simulink model "MSE_PLANT"  (R2025b)
settings: Solver=ode4  StartTime=0.0  StopTime=7  FixedStep=T  RelTol=1e-3  EnableMultiTasking=on
values from neighbouring files (symbols this model uses):
  b_sim = 0    [lab_1.m]    (also in lab_3.m)
  k_sim = 0    [lab_1.m]    (also in lab_3.m)
  Kt = Kt*motor_eff    (= 0.028)    [lab_1.m]    (also in lab_3.m)
  r = 0.01    [lab_1.m]    (also in lab_3.m)
  T = 0.001    [lab_1.m]    (also in lab_3.m)
undefined symbols (not defined in the file or in its folder): K_switch, Kd, Ki, Kp, National_Instruments, PCIe
libraries: sldrtlib x5, slpidlib x1
settings Model: ModifiedByFormat=C. Gokcek  SimulationMode=external  ExtModeTrigDuration=50  ExtModeWriteAllDataToWs=on  Creator=fdepi  LastModifiedBy=C. Gokcek
settings SolverCC: AlgebraicLoopSolver=TrustRegion
settings DataIOCC: SaveFormat=Array  SaveOutput=off  SignalLogging=off  DSMLogging=off  SaveTime=off  ReturnWorkspaceOutputs=off
settings OptimizationCC: ReuseModelBlockBuffer=off  ExpressionDepthLimit=2147483647.0  InitFltsAndDblsToZero=on  EfficientMapNaN2IntZero=off  LifeSpan=inf  SimCompilerOptimization=on
settings DebuggingCC: UnderspecifiedInitializationDetection=Classic  MergeDetectMultiDrivingBlocksExec=none  UnconnectedInputMsg=warning  UnconnectedOutputMsg=warning  UnconnectedLineMsg=warning  AllowSymbolicDim=off  StateNameClashWarn=warning  SFUnexpectedBacktrackingDiag=warning  SFNoUnconditionalDefaultTransitionDiag=warning  SFExecutionAtInitializationDiag=none  ArithmeticOperatorsInVariantConditions=warning
settings HardwareCC: ProdBitPerLong=64.0  ProdHWDeviceType=Intel->x86-64 (Linux 64)  TargetBitPerLong=64.0  TargetBitPerPointer=64.0  TargetIntDivRoundTo=Zero  TargetEndianess=LittleEndian  TargetWordSize=64.0  TargetHWDeviceType=Intel->x86-64
settings ModelReferenceCC: EnableRefExpFcnMdlSchedulingChecks=on  PropagateSignalLabelsOutOfModel=off
settings SFSimCC: SimUseLocalCustomCode=off  CustomCodeUndefinedFunction=UseInterfaceOnly
settings RTWCC: SystemTargetFile=sldrt.tlc  TemplateMakefile=sldrt.tmf  RTWVerbose=off  TLCAssert=on  RTWUseLocalCustomCode=off  RTWCompilerOptimization=on  GPUComputeCapability=3.5  DLArmComputeVersion=19.05  Description=Simulink Desktop Real-Time
settings CodeAppCC: GenerateComments=off  MaxIdLength=95.0  SimulinkBlockComments=off
settings SimulinkDesktopRealTimeCC: ExtModeTransport=0.0  ExtModeStaticAllocSize=1000000.0  TargetLibSuffix=_sldrt.a  TargetPreCompLibLocation=C:\Program Files\MATLAB\R2025b\toolbox\sldrt\lib\win64  TargetLangStandard=C89/C90 (ANSI)  MultiwordLength=2048.0  DynamicStringBufferSize=256.0  ParMdlRefBuildCompliant=on  PreserveMATLABNamespacesInGeneratedCode=on  SubcomponentCodeInterfacePackaging=Reusable function  SupportVariableSizeSignals=off
settings ConfigComp: CovMetricSettings=dw  CovSaveCumulativeToWorkspaceVar=on  CovSaveSingleToWorkspaceVar=on  CovExternalEMLEnable=off  CovSFcnEnable=off

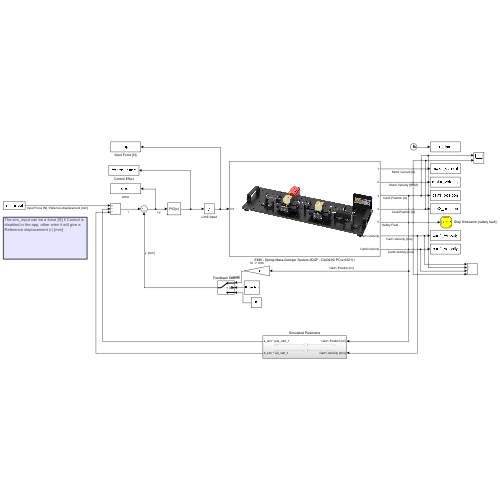
[thumbnail: Simulink's stored preview of the top-level diagram]
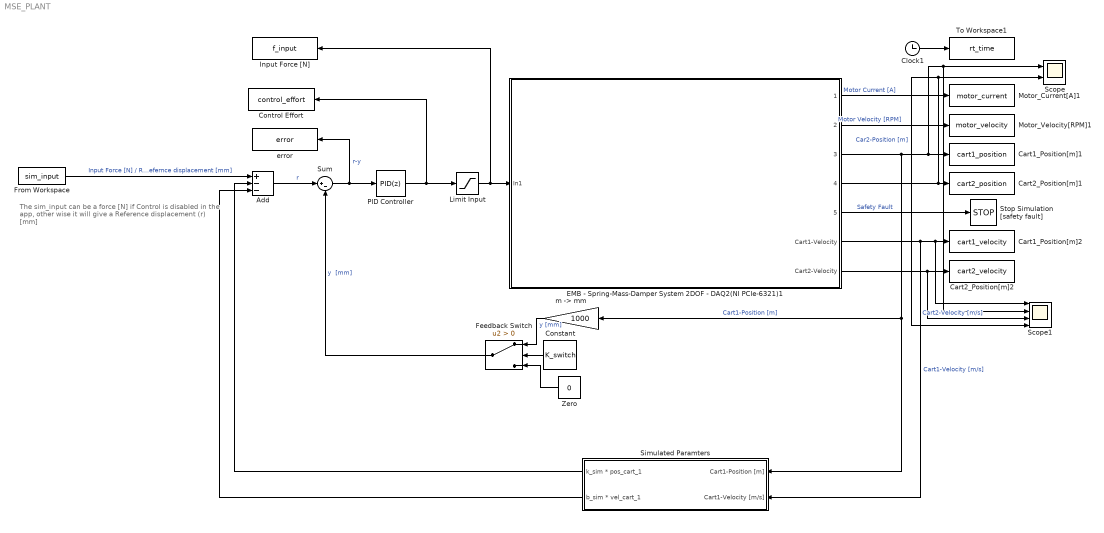
== system MSE_PLANT ==
  note: The sim_input can be a force [N] if Control is
      | disabled in the app, other wise it will give a
      | Reference displacement (r) [mm]
  Add : Sum  Inputs=+--
  Cart1_Position[m]1 : ToWorkspace  VariableName=cart1_position  SampleTime=-1
  Cart1_Position[m]2 : ToWorkspace  VariableName=cart1_velocity  SampleTime=-1
  Cart2_Position[m]1 : ToWorkspace  VariableName=cart2_position  SampleTime=-1
  Cart2_Position[m]2 : ToWorkspace  VariableName=cart2_velocity  SampleTime=-1
  Clock1 : Clock
  Constant : Constant  Value=K_switch
  Control Effort : ToWorkspace  VariableName=control_effort  SampleTime=-1
  EMB - Spring-Mass-Damper System 2DOF - DAQ2(NI PCIe-6321)1 : Subsystem
      mask Display: image('EMB-SMDS-2DOF.png');
  Feedback Switch : Switch  Criteria=u2 > Threshold  SaturateOnIntegerOverflow=off  InputSameDT=off
  From Workspace : FromWorkspace  VariableName=sim_input
  Input Force [N] : ToWorkspace  VariableName=f_input  SampleTime=-1
  Limit Input : Saturate  UpperLimit=10  LowerLimit=-10
  Motor_Current[A]1 : ToWorkspace  VariableName=motor_current  SampleTime=-1
  Motor_Velocity[RPM]1 : ToWorkspace  VariableName=motor_velocity  SampleTime=-1
  PID Controller : slpidlib/PID Controller  Controller=PID  Form=Parallel  TimeDomain=Discrete-time  UseExternalTs=off  SampleTime=T  IntegratorMethod=Forward Euler  FilterMethod=Forward Euler  ControllerParametersSource=internal  P=Kp  I=Ki  UseKiTs=off  D=Kd  UseExternalDerivativeSource=off  N=100  UseFilter=on  TunerSelectOption=Transfer Function Based (PID Tuner App)  InitialConditionSource=internal  InitialConditionForIntegrator=0  InitialConditionForFilter=0  DifferentiatorICPrevScaledInput=0  ExternalReset=none  TrackingMode=off  Kt=1  LimitOutput=off  SatLimitsSource=internal  UpperSaturationLimit=inf  LowerSaturationLimit=-inf  LinearizeAsGain=on  AntiWindupMode=none  Kb=1  LimitIntegrator=off  UpperIntegratorSaturationLimit=inf  LowerIntegratorSaturationLimit=-inf  POutMin=[]  POutMax=[]  IOutMin=[]  IOutMax=[]  DOutMin=[]  DOutMax=[]  NOutMin=[]  NOutMax=[]  SumOutMin=[]  SumOutMax=[]  SaturationOutMin=[]  SaturationOutMax=[]  PParamMin=[]  PParamMax=[]  IParamMin=[]  IParamMax=[]  DParamMin=[]  DParamMax=[]  NParamMin=[]  NParamMax=[]  KbParamMin=[]  KbParamMax=[]  KtParamMin=[]  KtParamMax=[]  KbOutMin=[]  KbOutMax=[]  KtOutMin=[]  KtOutMax=[]  IntegratorOutMin=[]  IntegratorOutMax=[]  FilterOutMin=[]  FilterOutMax=[]  SumI1OutMin=[]  SumI1OutMax=[]  SumI2OutMin=[]  SumI2OutMax=[]  SumI3OutMin=[]  SumI3OutMax=[]  SumI4OutMin=[]  SumI4OutMax=[]  SumDOutMin=[]  SumDOutMax=[]  DifferentiatorOutMin=[]  DifferentiatorOutMax=[]  FilterDiffOutCoefMin=[]  FilterDiffOutCoefMax=[]  ReciprocalOutMin=[]  ReciprocalOutMax=[]  SumDenOutMin=[]  SumDenOutMax=[]  SumNumOutMin=[]  SumNumOutMax=[]  DivideOutMin=[]  DivideOutMax=[]  UdiffTsProdOutMin=[]  UdiffTsProdOutMax=[]  NTsProdOutMin=[]  NTsProdOutMax=[]  UintegralTsProdOutMin=[]  UintegralTsProdOutMax=[]  UngainTsProdOutMin=[]  UngainTsProdOutMax=[]  ClampingZeroOutDataTypeStr=Inherit: Inherit via back propagation  ClampingZeroOutMin=[]  ClampingZeroOutMax=[]  FilterDenConstantOutDataTypeStr=Inherit: Inherit via back propagation  FilterDenConstantOutMin=[]  FilterDenConstantOutMax=[]  PCopyOutDataTypeStr=Inherit: Inherit via back propagation  PCopyOutMin=[]  PCopyOutMax=[]  NCopyOutDataTypeStr=Inherit: Inherit via back propagation  NCopyOutMin=[]  NCopyOutMax=[]  IntegratorContinuousStateAttributes=''  IntegratorStateMustResolveToSignalObject=off  IntegratorRTWStateStorageClass=Auto  FilterContinuousStateAttributes=''  FilterStateMustResolveToSignalObject=off  FilterRTWStateStorageClass=Auto  ParallelPVariant=InternalParameters  IdealPVariant=Disabled  IVariant=InternalParameters  DVariant=InternalParameters  IntegratorVariant=Discrete  SatVariant=Disabled  AWVariant=Passthrough  PCopyVariant=Disabled  TRVariant=Disabled  FdbkBlocksVariant=Forward  IdealPFdbkVariant=Disabled  SatFdbkVariant=Disabled  DerivativeFilterVariant=ForwardEulerFilter  NVariant=InternalParameters  NCopyVariant=Disabled  FilterICVariant=InternalICsFilter  IntegratorICVariant=InternalICs  ExternalResetVariant=Disabled  TRSumVariant=Passthrough  SumFdbkVariant=Disabled  SumVariant=Sum_PID  TsampFilterVariant=InternalTs  TsampNgainVariant=Passthrough  TsampIntegralVariant=Disabled_SignalSpec  ExternalSaturationOutDataTypeStr=Inherit: Same as second input  DerivativeSourceVariant=ErrorSignal  PreIntVariant=InternalPreInt
  Scope : Scope  NumInputPorts=2
      settings: ActiveDisplayYMinimum=-0.026393909411938546  ActiveDisplayYMaximum=0.050293861298803644
  Scope1 : Scope  NumInputPorts=4
      settings: ActiveDisplayYMinimum=-0.025542874999999996  ActiveDisplayYMaximum=0.029194124999999994
  Simulated Paramters : Subsystem
  Stop Simulation [safety fault] : Stop
  Sum : Sum  Inputs=|+-
  To Workspace1 : ToWorkspace  VariableName=rt_time  SampleTime=-1
  Zero : Constant  Value=0  OutDataTypeStr=Inherit: Inherit via back propagation
  error : ToWorkspace  VariableName=error  SampleTime=-1
  "m -> mm" : Gain  Gain=1000
  wires:
  EMB - Spring-Mass-Damper System 2DOF - DAQ2(NI PCIe-6321)1/7(Cart2-Velocity) -> Scope1/3, Cart2_Position[m]2/1  "Cart2-Velocity [m/s]"
  EMB - Spring-Mass-Damper System 2DOF - DAQ2(NI PCIe-6321)1/6(Cart1-Velocity) -> Simulated Paramters/2(Cart1-Velocity [m/s]), Scope1/1, Cart1_Position[m]2/1  "Cart1-Velocity [m/s]"
  EMB - Spring-Mass-Damper System 2DOF - DAQ2(NI PCIe-6321)1/1(1) -> Motor_Current[A]1/1  "Motor Current [A]"
  EMB - Spring-Mass-Damper System 2DOF - DAQ2(NI PCIe-6321)1/3(3) -> Simulated Paramters/1(Cart1-Position [m]), "m -> mm"/1, Scope/1, Scope1/2, Cart1_Position[m]1/1  "Cart1-Position [m]"
  EMB - Spring-Mass-Damper System 2DOF - DAQ2(NI PCIe-6321)1/2(2) -> Motor_Velocity[RPM]1/1  "Motor Velocity [RPM]"
  Limit Input/1 -> Input Force [N]/1, EMB - Spring-Mass-Damper System 2DOF - DAQ2(NI PCIe-6321)1/1(In1)
  EMB - Spring-Mass-Damper System 2DOF - DAQ2(NI PCIe-6321)1/5(5) -> Stop Simulation [safety fault]/1  "Safety Fault"
  EMB - Spring-Mass-Damper System 2DOF - DAQ2(NI PCIe-6321)1/4(4) -> Scope/2, Scope1/4, Cart2_Position[m]1/1  "Car2-Position [m]"
  Clock1/1 -> To Workspace1/1
  From Workspace/1 -> Add/1  "Input Force [N] / Refernce displacement [mm]"
  Simulated Paramters/1(k_sim * pos_cart_1) -> Add/2
  Simulated Paramters/2(b_sim * vel_cart_1) -> Add/3
  Zero/1 -> Feedback Switch/3
  "m -> mm"/1 -> Feedback Switch/1  "y [mm]"
  Add/1 -> Sum/1  "r"
  Sum/1 -> error/1, PID Controller/1  "r-y"
  PID Controller/1 -> Control Effort/1, Limit Input/1
  Feedback Switch/1 -> Sum/2  "y  [mm]"
  Constant/1 -> Feedback Switch/2

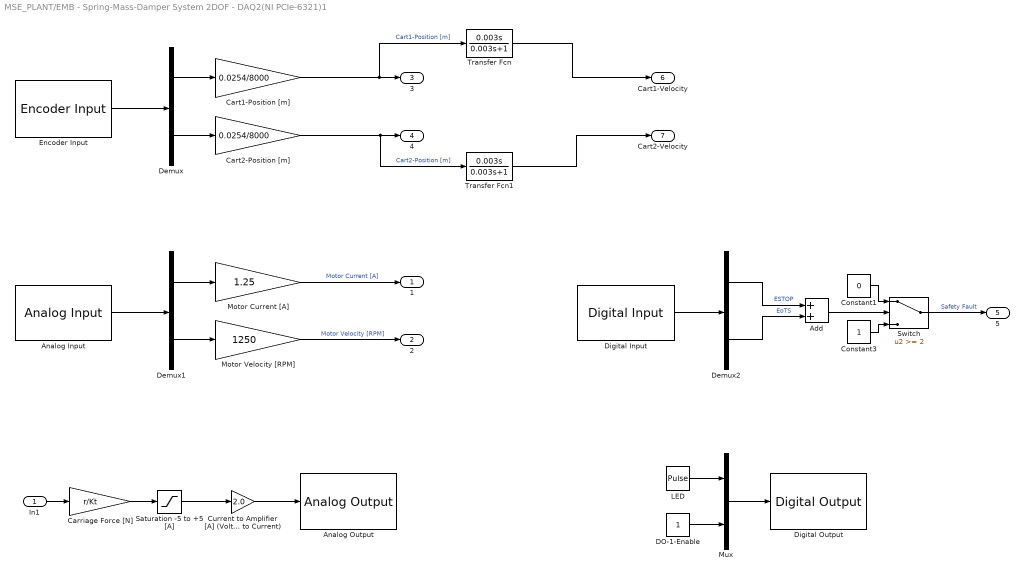
== system MSE_PLANT/EMB - Spring-Mass-Damper System 2DOF - DAQ2(NI PCIe-6321)1 ==
  In1 : Inport
  Add : Sum
  Analog Input : sldrtlib/Analog Input  SampleTime=T  MaxMissedTicks=10  ShowMissedTicks=off  YieldWhenWaiting=off  DrvName=National_Instruments/PCIe-6321  DrvAddress=4294967295  DrvOptions=[0 15 0 2 2 2 2]  Channels=[1,2]  RangeMode=1  VoltRange=2  DataType=1
      settings: AttributesFormatString=National Instruments\nPCIe-6321 [auto]
  Analog Output : sldrtlib/Analog Output  SampleTime=T  MaxMissedTicks=10  ShowMissedTicks=off  YieldWhenWaiting=off  DrvName=National_Instruments/PCIe-6321  DrvAddress=4294967295  DrvOptions=[0 15 0 2 2 2 2]  Channels=[1]  RangeMode=1  VoltRange=1  InitialValue=0  FinalValue=0
      settings: AttributesFormatString=National Instruments\nPCIe-6321 [auto]
  Carriage Force [N] : Gain  Gain=r/Kt
  Cart1-Position [m] : Gain  Gain=0.0254/8000
  Cart2-Position [m] : Gain  Gain=0.0254/8000
  Constant1 : Constant  Value=0
  Constant3 : Constant
  Current to Amplifier [A] (Voltage to Current) : Gain  Gain=2.0
  DO-1-Enable : Constant  OutDataTypeStr=double
  Demux : Demux  Outputs=2
  Demux1 : Demux  Outputs=2
  Demux2 : Demux  Outputs=2
  Digital Input : sldrtlib/Digital Input  SampleTime=T  MaxMissedTicks=10  ShowMissedTicks=off  YieldWhenWaiting=off  DrvName=National_Instruments/PCIe-6321  DrvAddress=4294967295  DrvOptions=[0 15 0 2 2 2 2]  Channels=[5,6]  BitMode=1  DataType=1
      settings: AttributesFormatString=National Instruments\nPCIe-6321 [auto]
  Digital Output : sldrtlib/Digital Output  SampleTime=T  MaxMissedTicks=10  ShowMissedTicks=off  YieldWhenWaiting=off  DrvName=National_Instruments/PCIe-6321  DrvAddress=4294967295  DrvOptions=[0 15 0 2 2 2 2]  Channels=[1,2]  BitMode=1  InitialValue=0  FinalValue=0
      settings: AttributesFormatString=National Instruments\nPCIe-6321 [auto]
  Encoder Input : sldrtlib/Encoder Input  SampleTime=T  MaxMissedTicks=10  ShowMissedTicks=off  YieldWhenWaiting=off  DrvName=National_Instruments/PCIe-6321  DrvAddress=4294967295  DrvOptions=[0 15 0 2 2 2 2]  Channels=[1,2]  QuadMode=3  IndexPulse=1  InputFilter=Inf  DataType=1
      settings: AttributesFormatString=National Instruments\nPCIe-6321 [auto]
  LED : DiscretePulseGenerator  PulseType=Time based  Period=0.5  PulseWidth=50
  Motor Current [A] : Gain  Gain=1.25
  Motor Velocity [RPM] : Gain  Gain=1250
  Mux : Mux  Inputs=2
  Saturation -5 to +5 [A] : Saturate  UpperLimit=5  LowerLimit=-5
  Switch : Switch  Threshold=2  SaturateOnIntegerOverflow=off  InputSameDT=off
  Transfer Fcn : TransferFcn  Numerator=[0.003 0]  Denominator=[0.003 1]
  Transfer Fcn1 : TransferFcn  Numerator=[0.003 0]  Denominator=[0.003 1]
  1 : Outport
  2 : Outport  Port=2
  3 : Outport  Port=3
  4 : Outport  Port=4
  5 : Outport  Port=5
  Cart1-Velocity : Outport  Port=6
  Cart2-Velocity : Outport  Port=7
  wires:
  Current to Amplifier [A] (Voltage to Current)/1 -> Analog Output/1
  Constant1/1 -> Switch/1
  Constant3/1 -> Switch/3
  DO-1-Enable/1 -> Mux/2
  Carriage Force [N]/1 -> Saturation -5 to +5 [A]/1
  Mux/1 -> Digital Output/1
  Motor Current [A]/1 -> 1/1  "Motor Current [A]"
  Cart1-Position [m]/1 -> Transfer Fcn/1, 3/1  "Cart1-Position [m]"
  Encoder Input/1 -> Demux/1
  Switch/1 -> 5/1  "Safety Fault"
  Demux1/2 -> Motor Velocity [RPM]/1
  Demux/2 -> Cart2-Position [m]/1
  Saturation -5 to +5 [A]/1 -> Current to Amplifier [A] (Voltage to Current)/1
  Demux1/1 -> Motor Current [A]/1
  Motor Velocity [RPM]/1 -> 2/1  "Motor Velocity [RPM]"
  Demux2/2 -> Add/2  "EoTS"
  Demux/1 -> Cart1-Position [m]/1
  Digital Input/1 -> Demux2/1
  Demux2/1 -> Add/1  "ESTOP"
  Analog Input/1 -> Demux1/1
  LED/1 -> Mux/1
  Add/1 -> Switch/2
  In1/1 -> Carriage Force [N]/1
  Cart2-Position [m]/1 -> Transfer Fcn1/1, 4/1  "Cart2-Position [m]"
  Transfer Fcn/1 -> Cart1-Velocity/1
  Transfer Fcn1/1 -> Cart2-Velocity/1

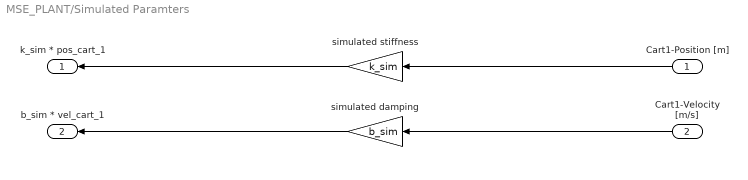
== system MSE_PLANT/Simulated Paramters ==
  Cart1-Position [m] : Inport
  Cart1-Velocity [m/s] : Inport  Port=2
  simulated damping : Gain  Gain=b_sim
  simulated stiffness : Gain  Gain=k_sim
  k_sim * pos_cart_1 : Outport
  b_sim * vel_cart_1 : Outport  Port=2
  wires:
  simulated damping/1 -> b_sim * vel_cart_1/1
  Cart1-Velocity [m/s]/1 -> simulated damping/1
  simulated stiffness/1 -> k_sim * pos_cart_1/1
  Cart1-Position [m]/1 -> simulated stiffness/1
